simulink model "avg_speed"  (R2023b)
settings: Solver=FixedStepDiscrete  StartTime=0.0  StopTime=10.0  FixedStep=0.01  RelTol=1e-3
model workspace (MAT data in the model file):
  threshold = Simulink.Parameter
  threshold.Value = 25
  threshold.DataType = 'single'
  threshold.Complexity = 'real'
  threshold.Dimensions = [1 1]
settings Model: Creator=developer  LastModifiedBy=developer
settings OptimizationCC: DefaultParameterBehavior=Inlined  EnhancedBackFolding=on  PassReuseOutputArgsAs=Individual arguments  ZeroExternalMemoryAtStartup=off  ZeroInternalMemoryAtStartup=off  OptimizeBlockOrder=speed  DifferentSizesBufferReuse=on  OptimizationCustomize=off  EfficientTunableParamExpr=on
settings DebuggingCC: ParameterTunabilityLossMsg=error  BusObjectLabelMismatch=error
settings SFSimCC: MATLABDynamicMemAlloc=off
settings RTWCC: Description=Embedded Coder  SystemTargetFile=ert.tlc  TemplateMakefile=ert_default_tmf
settings CodeAppCC: ForceParamTrailComments=on  IgnoreCustomStorageClasses=off  OperatorAnnotations=on  SimulinkDataObjDesc=on  SFDataObjDesc=on  InsertBlockDesc=on
settings ERTTargetCC: TargetLangStandard=C99 (ISO)  GenerateSampleERTMain=on  InlinedParameterPlacement=NonHierarchical  ERTCustomFileTemplate=example_file_process.tlc

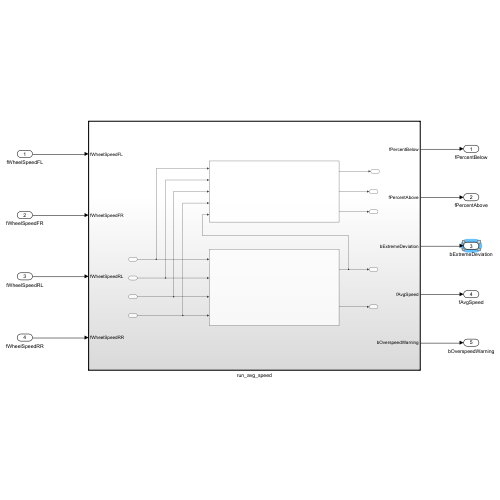
[thumbnail: Simulink's stored preview of the top-level diagram]
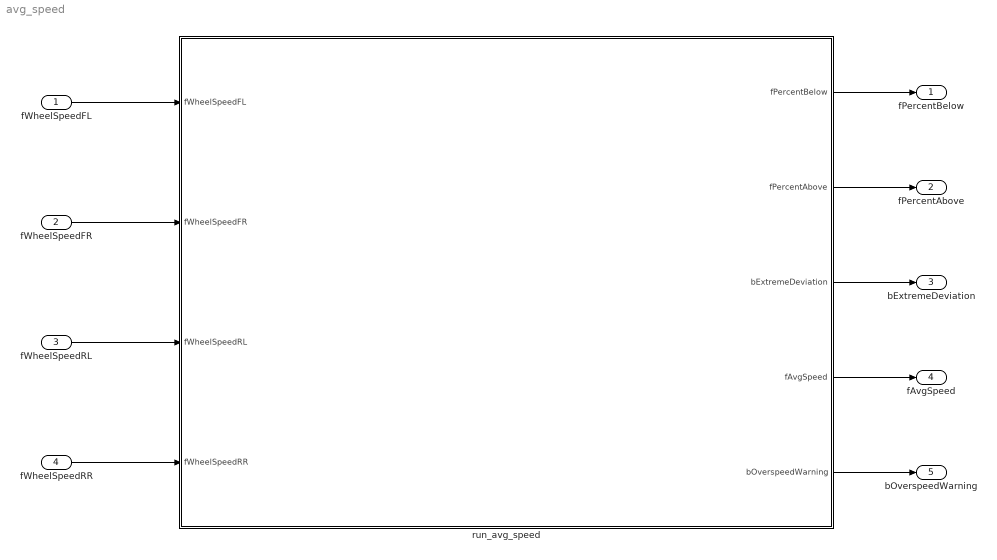
== system avg_speed ==
  fWheelSpeedFL : Inport
  fWheelSpeedFR : Inport  Port=2
  fWheelSpeedRL : Inport  Port=3
  fWheelSpeedRR : Inport  Port=4
  run_avg_speed : Subsystem  TreatAsAtomicUnit=on
  fPercentBelow : Outport
  fPercentAbove : Outport  Port=2
  bExtremeDeviation : Outport  Port=3  OutDataTypeStr=boolean
  fAvgSpeed : Outport  Port=4
  bOverspeedWarning : Outport  Port=5
  wires:
  run_avg_speed/4(fAvgSpeed) -> fAvgSpeed/1
  run_avg_speed/3(bExtremeDeviation) -> bExtremeDeviation/1
  run_avg_speed/2(fPercentAbove) -> fPercentAbove/1
  fWheelSpeedFL/1 -> run_avg_speed/1(fWheelSpeedFL)
  fWheelSpeedFR/1 -> run_avg_speed/2(fWheelSpeedFR)
  fWheelSpeedRL/1 -> run_avg_speed/3(fWheelSpeedRL)
  fWheelSpeedRR/1 -> run_avg_speed/4(fWheelSpeedRR)
  run_avg_speed/1(fPercentBelow) -> fPercentBelow/1
  run_avg_speed/5(bOverspeedWarning) -> bOverspeedWarning/1

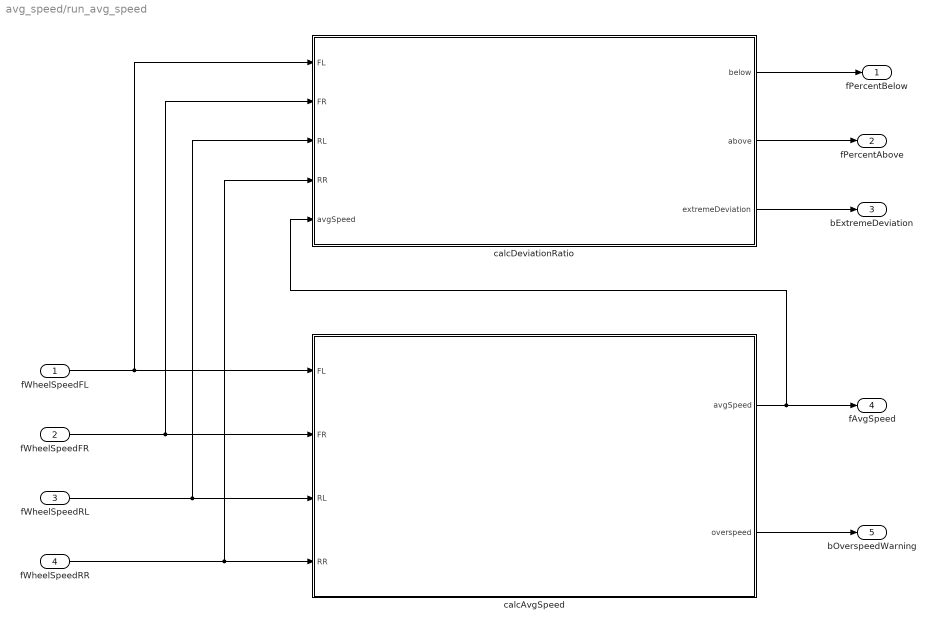
== system avg_speed/run_avg_speed ==
  fWheelSpeedFL : Inport
  fWheelSpeedFR : Inport  Port=2
  fWheelSpeedRL : Inport  Port=3
  fWheelSpeedRR : Inport  Port=4
  calcAvgSpeed : Subsystem  TreatAsAtomicUnit=on
  calcDeviationRatio : Subsystem  TreatAsAtomicUnit=on
  fPercentBelow : Outport
  fPercentAbove : Outport  Port=2
  bExtremeDeviation : Outport  Port=3
  fAvgSpeed : Outport  Port=4
  bOverspeedWarning : Outport  Port=5
  wires:
  fWheelSpeedRR/1 -> calcAvgSpeed/4(RR), calcDeviationRatio/4(RR)
  fWheelSpeedFL/1 -> calcDeviationRatio/1(FL), calcAvgSpeed/1(FL)
  fWheelSpeedRL/1 -> calcAvgSpeed/3(RL), calcDeviationRatio/3(RL)
  calcAvgSpeed/2(overspeed) -> bOverspeedWarning/1
  fWheelSpeedFR/1 -> calcAvgSpeed/2(FR), calcDeviationRatio/2(FR)
  calcDeviationRatio/2(above) -> fPercentAbove/1
  calcAvgSpeed/1(avgSpeed) -> fAvgSpeed/1, calcDeviationRatio/5(avgSpeed)
  calcDeviationRatio/1(below) -> fPercentBelow/1
  calcDeviationRatio/3(extremeDeviation) -> bExtremeDeviation/1

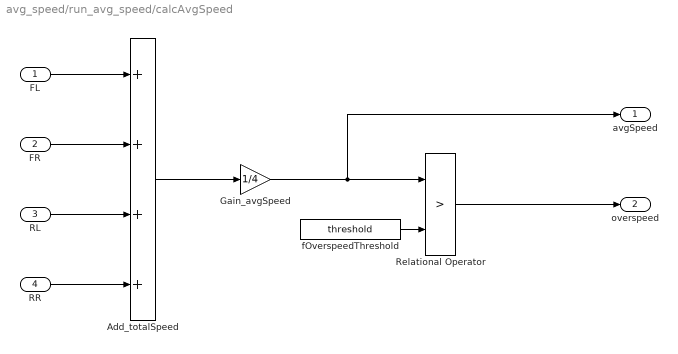
== system avg_speed/run_avg_speed/calcAvgSpeed ==
  FL : Inport
  FR : Inport  Port=2
  RL : Inport  Port=3
  RR : Inport  Port=4
  Add_totalSpeed : Sum  Inputs=++++
  Gain_avgSpeed : Gain  Gain=1/4
  Relational Operator : RelationalOperator  Operator=>  OutDataTypeStr=boolean  RndMeth=Simplest  InputSameDT=off
  fOverspeedThreshold : Constant  Value=threshold
  avgSpeed : Outport
  overspeed : Outport  Port=2
  wires:
  fOverspeedThreshold/1 -> Relational Operator/2
  Gain_avgSpeed/1 -> avgSpeed/1, Relational Operator/1
  RL/1 -> Add_totalSpeed/3
  FR/1 -> Add_totalSpeed/2
  Add_totalSpeed/1 -> Gain_avgSpeed/1
  Relational Operator/1 -> overspeed/1
  RR/1 -> Add_totalSpeed/4
  FL/1 -> Add_totalSpeed/1

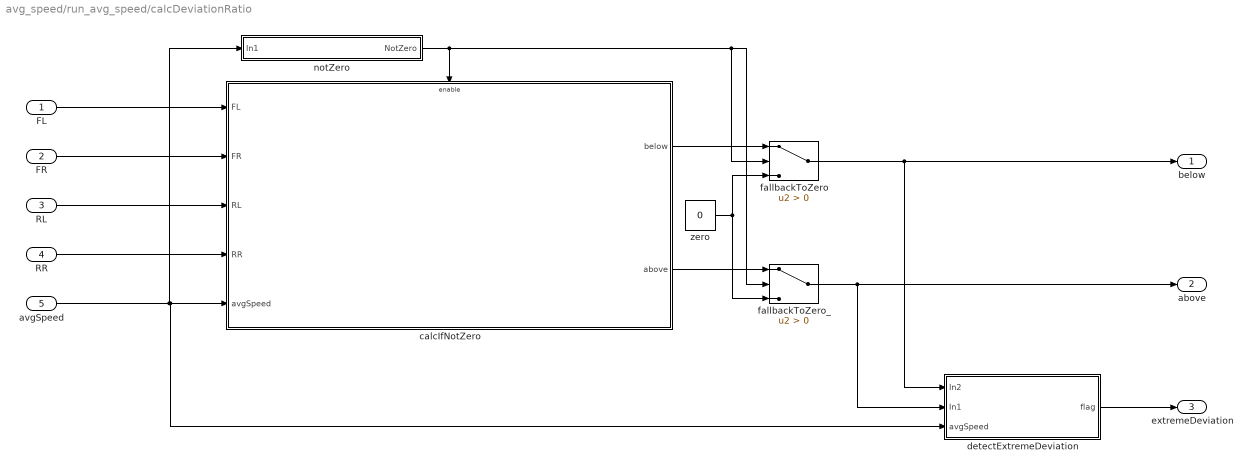
== system avg_speed/run_avg_speed/calcDeviationRatio ==
  FL : Inport
  FR : Inport  Port=2
  RL : Inport  Port=3
  RR : Inport  Port=4
  avgSpeed : Inport  Port=5
  calcIfNotZero : Subsystem
      settings: RTWSystemCode=Nonreusable function  RTWFcnNameOpts=Use subsystem name
  detectExtremeDeviation : Subsystem
  fallbackToZero : Switch  Criteria=u2 > Threshold  SaturateOnIntegerOverflow=off  InputSameDT=off
  fallbackToZero_ : Switch  Criteria=u2 > Threshold  SaturateOnIntegerOverflow=off  InputSameDT=off
  notZero : Subsystem
  zero : Constant  Value=0
  below : Outport
  above : Outport  Port=2
  extremeDeviation : Outport  Port=3
  wires:
  notZero/1(NotZero) -> calcIfNotZero/Enable, fallbackToZero_/2, fallbackToZero/2
  RR/1 -> calcIfNotZero/4(RR)
  calcIfNotZero/1(below) -> fallbackToZero/1
  calcIfNotZero/2(above) -> fallbackToZero_/1
  avgSpeed/1 -> notZero/1(In1), detectExtremeDeviation/3(avgSpeed), calcIfNotZero/5(avgSpeed)
  FR/1 -> calcIfNotZero/2(FR)
  zero/1 -> fallbackToZero_/3, fallbackToZero/3
  FL/1 -> calcIfNotZero/1(FL)
  RL/1 -> calcIfNotZero/3(RL)
  fallbackToZero/1 -> detectExtremeDeviation/1(In2), below/1
  fallbackToZero_/1 -> detectExtremeDeviation/2(In1), above/1
  detectExtremeDeviation/1(flag) -> extremeDeviation/1

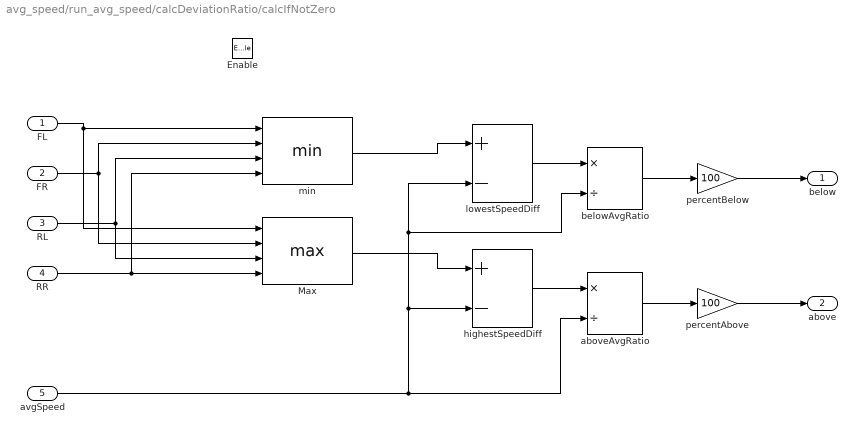
== system avg_speed/run_avg_speed/calcDeviationRatio/calcIfNotZero ==
  FL : Inport
  FR : Inport  Port=2
  RL : Inport  Port=3
  RR : Inport  Port=4
  avgSpeed : Inport  Port=5
  Enable : EnablePort
  Max : MinMax  Function=max  Inputs=4
  aboveAvgRatio : Product  Inputs=*/
  belowAvgRatio : Product  Inputs=*/
  highestSpeedDiff : Sum  Inputs=+-
  lowestSpeedDiff : Sum  Inputs=+-
  min : MinMax  Inputs=4
  percentAbove : Gain  Gain=100
  percentBelow : Gain  Gain=100
  below : Outport
  above : Outport  Port=2
  wires:
  min/1 -> lowestSpeedDiff/1
  RL/1 -> min/3, Max/3
  FL/1 -> Max/1, min/1
  RR/1 -> min/4, Max/4
  FR/1 -> Max/2, min/2
  percentAbove/1 -> above/1
  Max/1 -> highestSpeedDiff/1
  lowestSpeedDiff/1 -> belowAvgRatio/1
  belowAvgRatio/1 -> percentBelow/1
  highestSpeedDiff/1 -> aboveAvgRatio/1
  aboveAvgRatio/1 -> percentAbove/1
  avgSpeed/1 -> aboveAvgRatio/2, belowAvgRatio/2, lowestSpeedDiff/2, highestSpeedDiff/2
  percentBelow/1 -> below/1

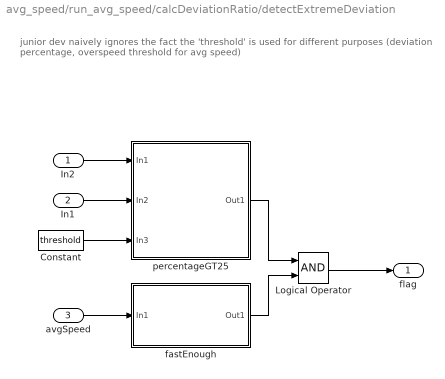
== system avg_speed/run_avg_speed/calcDeviationRatio/detectExtremeDeviation ==
  note: junior dev naively ignores the fact the 'threshold' is used for different purposes (deviation percentage, overspeed threshold for avg speed)
  In2 : Inport
  In1 : Inport  Port=2
  avgSpeed : Inport  Port=3
  Constant : Constant  Value=threshold
  Logical Operator : Logic  AllPortsSameDT=off  OutDataTypeStr=boolean
  fastEnough : Subsystem
  percentageGT25 : Subsystem
  flag : Outport
  wires:
  In2/1 -> percentageGT25/1(In1)
  Logical Operator/1 -> flag/1
  In1/1 -> percentageGT25/2(In2)
  Constant/1 -> percentageGT25/3(In3)
  avgSpeed/1 -> fastEnough/1(In1)
  percentageGT25/1(Out1) -> Logical Operator/1
  fastEnough/1(Out1) -> Logical Operator/2

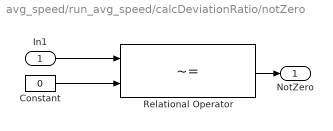
== system avg_speed/run_avg_speed/calcDeviationRatio/notZero ==
  In1 : Inport
  Constant : Constant  Value=0
  Relational Operator : RelationalOperator  Operator=~=  OutDataTypeStr=boolean  RndMeth=Simplest  InputSameDT=off
  NotZero : Outport
  wires:
  Constant/1 -> Relational Operator/2
  Relational Operator/1 -> NotZero/1
  In1/1 -> Relational Operator/1

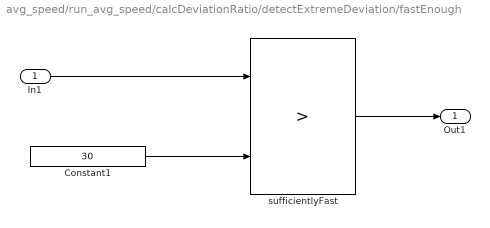
== system avg_speed/run_avg_speed/calcDeviationRatio/detectExtremeDeviation/fastEnough ==
  In1 : Inport
  Constant1 : Constant  Value=30
  sufficientlyFast : RelationalOperator  Operator=>  OutDataTypeStr=boolean  RndMeth=Simplest  InputSameDT=off
  Out1 : Outport
  wires:
  Constant1/1 -> sufficientlyFast/2
  In1/1 -> sufficientlyFast/1
  sufficientlyFast/1 -> Out1/1

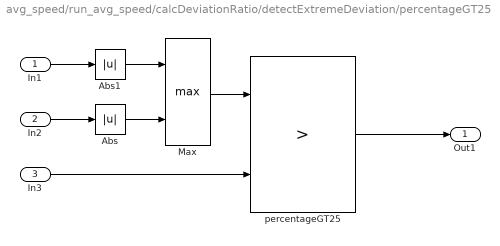
== system avg_speed/run_avg_speed/calcDeviationRatio/detectExtremeDeviation/percentageGT25 ==
  In1 : Inport
  In2 : Inport  Port=2
  In3 : Inport  Port=3
  Abs : Abs  SaturateOnIntegerOverflow=off
  Abs1 : Abs  SaturateOnIntegerOverflow=off
  Max : MinMax  Function=max  Inputs=2
  percentageGT25 : RelationalOperator  Operator=>  OutDataTypeStr=boolean  RndMeth=Simplest  InputSameDT=off
  Out1 : Outport
  wires:
  Max/1 -> percentageGT25/1
  Abs1/1 -> Max/1
  percentageGT25/1 -> Out1/1
  In3/1 -> percentageGT25/2
  Abs/1 -> Max/2
  In2/1 -> Abs/1
  In1/1 -> Abs1/1
